simulink subsystem "Piero"  (R2023b)
settings: Solver=VariableStepAuto  StartTime=0.0  StopTime=10.0  RelTol=1e-3
settings Model: Creator=Usuario  LastModifiedBy=Usuario

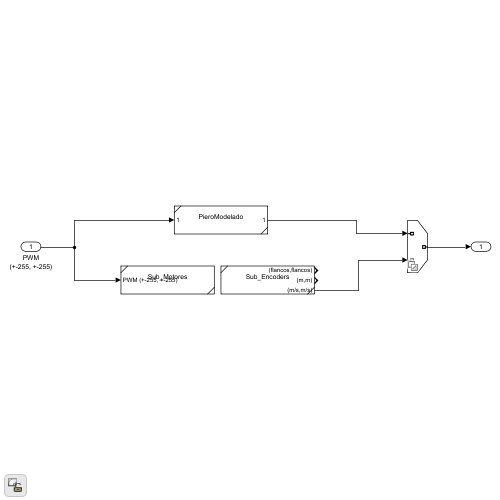
[thumbnail: Simulink's stored preview of the top-level diagram]
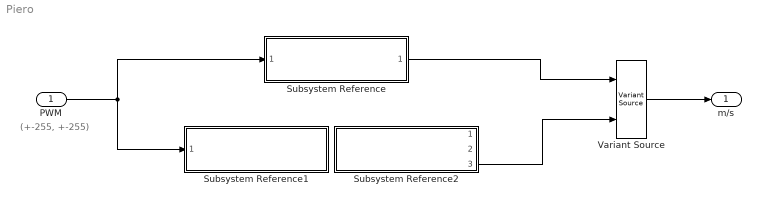
== system Piero ==
  note: (+-255, +-255)
  PWM : Inport
  Subsystem Reference : Subsystem  ReferencedSubsystem=PieroModelado
  Subsystem Reference1 : Subsystem  ReferencedSubsystem=Sub_Motores
  Subsystem Reference2 : Subsystem  ReferencedSubsystem=Sub_Encoders
  Variant Source : VariantSource  VariantControlMode=sim codegen switching
  m/s : Outport
  wires:
  PWM/1 -> Subsystem Reference/1, Subsystem Reference1/1
  Subsystem Reference/1 -> Variant Source/1
  Subsystem Reference2/3 -> Variant Source/2
  Variant Source/1 -> m/s/1
